simulink model "PMSMController"  (R2021a)
settings: Solver=FixedStepDiscrete  StartTime=0.0  StopTime=T_end  FixedStep=mask_Ts  RelTol=1e-3
values from neighbouring files (symbols this model uses):
  f_w = 50    [speedControlInit.m]
  Iq_max = 200    [speedControlInit.m]
  mask_Kaw = mask_Kis/mask_Kps    (= 1.25e-06)    [speedControlInit.m]
  mask_Kid = omega_ib*mask_R_s    (= 212.057504117)    [speedControlInit.m]
  mask_Kiq = omega_ib*mask_R_s    (= 212.057504117)    [speedControlInit.m]
  mask_Kis = omega_sb*B    (= 1.1780972451e-05)    [speedControlInit.m]
  mask_Kpd = omega_ib*mask_Ld    (= 0.249285377062)    [speedControlInit.m]
  mask_Kpq = omega_ib*mask_Lq    (= 0.249285377062)    [speedControlInit.m]
  mask_Kps = omega_sb*J    (= 9.42477796077)    [speedControlInit.m]
  mask_Kt = 0.126    [speedControlInit.m]
  mask_lambda_pm = mask_Kt/((3/2)*mask_p)    (= 0.0105)    [speedControlInit.m]
  mask_Ld = 52.9e-6    (= 5.29e-05)    [speedControlInit.m]
  mask_Lq = 52.9e-6    (= 5.29e-05)    [speedControlInit.m]
  mask_p = 8    [speedControlInit.m]
  mask_Ts = 1/10000    (= 0.0001)    [speedControlInit.m]
  mask_VDC = 250    [speedControlInit.m]
libraries: pid_lib x3
settings Model: Creator=Nishanth  LastModifiedBy=Nishanth
settings SolverCC: AlgebraicLoopSolver=TrustRegion
settings DataIOCC: SaveOutput=off  SaveTime=off
settings OptimizationCC: DefaultParameterBehavior=Inlined  EnhancedBackFolding=on  PassReuseOutputArgsAs=Individual arguments  ZeroExternalMemoryAtStartup=off  ZeroInternalMemoryAtStartup=off  NoFixptDivByZeroProtection=on  EfficientFloat2IntCast=on  OptimizeBlockOrder=speed  DifferentSizesBufferReuse=on  OptimizationCustomize=off  EfficientTunableParamExpr=on
settings DebuggingCC: ParameterTunabilityLossMsg=error  SFMachineParentedDataDiag=warning
settings SFSimCC: MATLABDynamicMemAlloc=off
settings RTWCC: SystemTargetFile=ert.tlc  GenCodeOnly=on  TemplateMakefile=ert_default_tmf  GenerateReport=on  LaunchReport=on  GenerateCodeMetricsReport=on
settings CodeAppCC: ForceParamTrailComments=on  IgnoreCustomStorageClasses=off  OperatorAnnotations=on  SimulinkDataObjDesc=on  SFDataObjDesc=on  InsertBlockDesc=on
settings ERTTargetCC: TargetLangStandard=C99 (ISO)  SupportNonFinite=off  RemoveResetFunc=off  InlinedParameterPlacement=NonHierarchical  ERTCustomFileTemplate=example_file_process.tlc

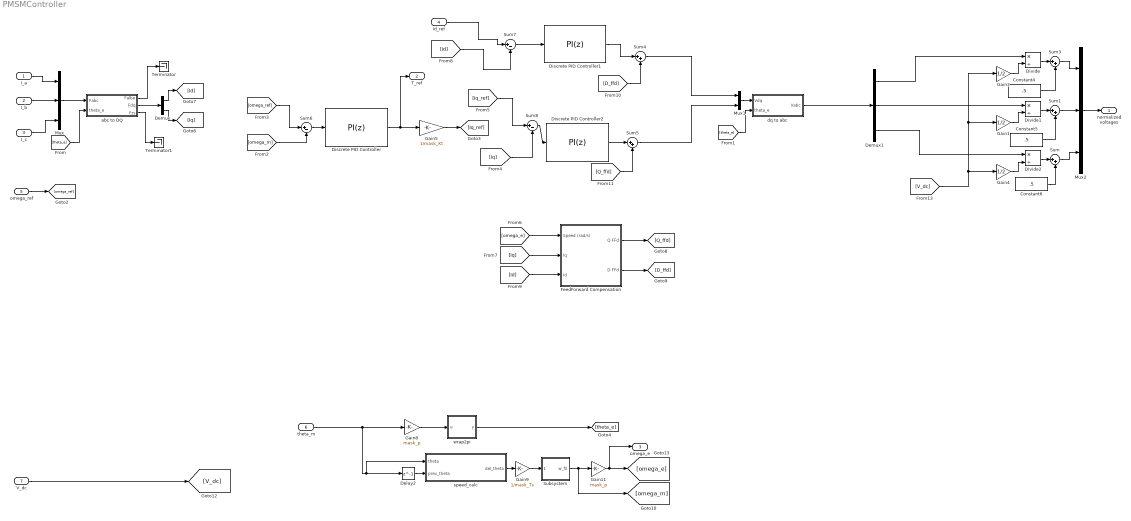
== system PMSMController ==
  I_a : Inport  OutDataTypeStr=double  PortDimensions=1
  I_b : Inport  Port=2  OutDataTypeStr=double  PortDimensions=1
  I_c : Inport  Port=3  OutDataTypeStr=double  PortDimensions=1
  Id_ref : Inport  Port=4  OutDataTypeStr=double  PortDimensions=1
  omega_ref : Inport  Port=5  OutDataTypeStr=double  PortDimensions=1
  theta_m : Inport  Port=6  OutDataTypeStr=double  PortDimensions=1
  V_dc : Inport  Port=7  OutDataTypeStr=double  PortDimensions=1
  Constant4 : Constant  Value=.5
  Constant5 : Constant  Value=.5
  Constant6 : Constant  Value=.5
  Delay2 : Delay  DelayLength=1
  Demux : Demux  Outputs=2
  Demux1 : Demux  Outputs=3
  Discrete PID Controller : pid_lib/PID Controller  Controller=PI  Form=Parallel  TimeDomain=Discrete-time  UseExternalTs=off  SampleTime=-1  IntegratorMethod=Forward Euler  FilterMethod=Forward Euler  ControllerParametersSource=internal  P=mask_Kps  I=mask_Kis  D=0  UseFilter=off  N=100  TunerSelectOption=Transfer Function Based (PID Tuner App)  ZeroCross=off  InitialConditionSource=internal  InitialConditionForIntegrator=0  InitialConditionForFilter=0  DifferentiatorICPrevScaledInput=0  ExternalReset=none  TrackingMode=off  Kt=1  LimitOutput=on  SatLimitsSource=internal  UpperSaturationLimit=Iq_max*mask_Kt  LowerSaturationLimit=-Iq_max*mask_Kt  LinearizeAsGain=off  AntiWindupMode=back-calculation  Kb=mask_Kaw  POutMin=[]  POutMax=[]  IOutMin=[]  IOutMax=[]  DOutMin=[]  DOutMax=[]  NOutMin=[]  NOutMax=[]  SumOutMin=[]  SumOutMax=[]  SaturationOutMin=[]  SaturationOutMax=[]  PParamMin=[]  PParamMax=[]  IParamMin=[]  IParamMax=[]  DParamMin=[]  DParamMax=[]  NParamMin=[]  NParamMax=[]  KbParamMin=[]  KbParamMax=[]  KtParamMin=[]  KtParamMax=[]  KbOutMin=[]  KbOutMax=[]  KtOutMin=[]  KtOutMax=[]  IntegratorOutMin=[]  IntegratorOutMax=[]  FilterOutMin=[]  FilterOutMax=[]  SumI1OutMin=[]  SumI1OutMax=[]  SumI2OutMin=[]  SumI2OutMax=[]  SumI3OutMin=[]  SumI3OutMax=[]  SumI4OutMin=[]  SumI4OutMax=[]  SumDOutMin=[]  SumDOutMax=[]  DifferentiatorOutMin=[]  DifferentiatorOutMax=[]  FilterDiffOutCoefMin=[]  FilterDiffOutCoefMax=[]  ReciprocalOutMin=[]  ReciprocalOutMax=[]  SumDenOutMin=[]  SumDenOutMax=[]  SumNumOutMin=[]  SumNumOutMax=[]  DivideOutMin=[]  DivideOutMax=[]  UdiffTsProdOutMin=[]  UdiffTsProdOutMax=[]  NTsProdOutMin=[]  NTsProdOutMax=[]  UintegralTsProdOutMin=[]  UintegralTsProdOutMax=[]  UngainTsProdOutMin=[]  UngainTsProdOutMax=[]  IntegratorContinuousStateAttributes=''  IntegratorStateMustResolveToSignalObject=off  IntegratorRTWStateStorageClass=Auto  FilterContinuousStateAttributes=''  FilterStateMustResolveToSignalObject=off  FilterRTWStateStorageClass=Auto  ParallelPVariant=InternalParameters  IdealPVariant=Disabled  IVariant=InternalParameters  DVariant=Disabled  IntegratorVariant=Discrete  SatVariant=Enabled  AWVariant=BackCalculation  PCopyVariant=Disabled  TRVariant=Disabled  FdbkBlocksVariant=Forward  IdealPFdbkVariant=Disabled  SatFdbkVariant=Disabled  DerivativeFilterVariant=Disabled  NVariant=Disabled  NCopyVariant=Disabled_SignalSpec  FilterICVariant=Disabled  IntegratorICVariant=InternalICs  ExternalResetVariant=Disabled  TRSumVariant=Passthrough  SumFdbkVariant=Disabled  SumVariant=Sum_PI  TsampFilterVariant=InternalTs  TsampNgainVariant=Passthrough  TsampIntegralVariant=Passthrough  ExternalSaturationOutDataTypeStr=Inherit: Same as second input
  Discrete PID Controller1 : pid_lib/PID Controller  Controller=PI  Form=Parallel  TimeDomain=Discrete-time  UseExternalTs=off  SampleTime=-1  IntegratorMethod=Forward Euler  FilterMethod=Forward Euler  ControllerParametersSource=internal  P=mask_Kpd  I=mask_Kid  D=0  UseFilter=off  N=100  TunerSelectOption=Transfer Function Based (PID Tuner App)  ZeroCross=off  InitialConditionSource=internal  InitialConditionForIntegrator=0  InitialConditionForFilter=0  DifferentiatorICPrevScaledInput=0  ExternalReset=none  TrackingMode=off  Kt=1  LimitOutput=off  SatLimitsSource=internal  UpperSaturationLimit=mask_VDC/2  LowerSaturationLimit=-mask_VDC/2  LinearizeAsGain=off  AntiWindupMode=back-calculation  Kb=mask_Kaw  POutMin=[]  POutMax=[]  IOutMin=[]  IOutMax=[]  DOutMin=[]  DOutMax=[]  NOutMin=[]  NOutMax=[]  SumOutMin=[]  SumOutMax=[]  SaturationOutMin=[]  SaturationOutMax=[]  PParamMin=[]  PParamMax=[]  IParamMin=[]  IParamMax=[]  DParamMin=[]  DParamMax=[]  NParamMin=[]  NParamMax=[]  KbParamMin=[]  KbParamMax=[]  KtParamMin=[]  KtParamMax=[]  KbOutMin=[]  KbOutMax=[]  KtOutMin=[]  KtOutMax=[]  IntegratorOutMin=[]  IntegratorOutMax=[]  FilterOutMin=[]  FilterOutMax=[]  SumI1OutMin=[]  SumI1OutMax=[]  SumI2OutMin=[]  SumI2OutMax=[]  SumI3OutMin=[]  SumI3OutMax=[]  SumI4OutMin=[]  SumI4OutMax=[]  SumDOutMin=[]  SumDOutMax=[]  DifferentiatorOutMin=[]  DifferentiatorOutMax=[]  FilterDiffOutCoefMin=[]  FilterDiffOutCoefMax=[]  ReciprocalOutMin=[]  ReciprocalOutMax=[]  SumDenOutMin=[]  SumDenOutMax=[]  SumNumOutMin=[]  SumNumOutMax=[]  DivideOutMin=[]  DivideOutMax=[]  UdiffTsProdOutMin=[]  UdiffTsProdOutMax=[]  NTsProdOutMin=[]  NTsProdOutMax=[]  UintegralTsProdOutMin=[]  UintegralTsProdOutMax=[]  UngainTsProdOutMin=[]  UngainTsProdOutMax=[]  IntegratorContinuousStateAttributes=''  IntegratorStateMustResolveToSignalObject=off  IntegratorRTWStateStorageClass=Auto  FilterContinuousStateAttributes=''  FilterStateMustResolveToSignalObject=off  FilterRTWStateStorageClass=Auto  ParallelPVariant=InternalParameters  IdealPVariant=Disabled  IVariant=InternalParameters  DVariant=Disabled  IntegratorVariant=Discrete  SatVariant=Disabled  AWVariant=Passthrough  PCopyVariant=Disabled  TRVariant=Disabled  FdbkBlocksVariant=Forward  IdealPFdbkVariant=Disabled  SatFdbkVariant=Disabled  DerivativeFilterVariant=Disabled  NVariant=Disabled  NCopyVariant=Disabled_SignalSpec  FilterICVariant=Disabled  IntegratorICVariant=InternalICs  ExternalResetVariant=Disabled  TRSumVariant=Passthrough  SumFdbkVariant=Disabled  SumVariant=Sum_PI  TsampFilterVariant=InternalTs  TsampNgainVariant=Passthrough  TsampIntegralVariant=Passthrough  ExternalSaturationOutDataTypeStr=Inherit: Same as second input
  Discrete PID Controller2 : pid_lib/PID Controller  Controller=PI  Form=Parallel  TimeDomain=Discrete-time  UseExternalTs=off  SampleTime=-1  IntegratorMethod=Forward Euler  FilterMethod=Forward Euler  ControllerParametersSource=internal  P=mask_Kpq  I=mask_Kiq  D=0  UseFilter=off  N=100  TunerSelectOption=Transfer Function Based (PID Tuner App)  ZeroCross=off  InitialConditionSource=internal  InitialConditionForIntegrator=0  InitialConditionForFilter=0  DifferentiatorICPrevScaledInput=0  ExternalReset=none  TrackingMode=off  Kt=1  LimitOutput=off  SatLimitsSource=internal  UpperSaturationLimit=mask_VDC/2  LowerSaturationLimit=-mask_VDC/2  LinearizeAsGain=off  AntiWindupMode=back-calculation  Kb=mask_Kaw  POutMin=[]  POutMax=[]  IOutMin=[]  IOutMax=[]  DOutMin=[]  DOutMax=[]  NOutMin=[]  NOutMax=[]  SumOutMin=[]  SumOutMax=[]  SaturationOutMin=[]  SaturationOutMax=[]  PParamMin=[]  PParamMax=[]  IParamMin=[]  IParamMax=[]  DParamMin=[]  DParamMax=[]  NParamMin=[]  NParamMax=[]  KbParamMin=[]  KbParamMax=[]  KtParamMin=[]  KtParamMax=[]  KbOutMin=[]  KbOutMax=[]  KtOutMin=[]  KtOutMax=[]  IntegratorOutMin=[]  IntegratorOutMax=[]  FilterOutMin=[]  FilterOutMax=[]  SumI1OutMin=[]  SumI1OutMax=[]  SumI2OutMin=[]  SumI2OutMax=[]  SumI3OutMin=[]  SumI3OutMax=[]  SumI4OutMin=[]  SumI4OutMax=[]  SumDOutMin=[]  SumDOutMax=[]  DifferentiatorOutMin=[]  DifferentiatorOutMax=[]  FilterDiffOutCoefMin=[]  FilterDiffOutCoefMax=[]  ReciprocalOutMin=[]  ReciprocalOutMax=[]  SumDenOutMin=[]  SumDenOutMax=[]  SumNumOutMin=[]  SumNumOutMax=[]  DivideOutMin=[]  DivideOutMax=[]  UdiffTsProdOutMin=[]  UdiffTsProdOutMax=[]  NTsProdOutMin=[]  NTsProdOutMax=[]  UintegralTsProdOutMin=[]  UintegralTsProdOutMax=[]  UngainTsProdOutMin=[]  UngainTsProdOutMax=[]  IntegratorContinuousStateAttributes=''  IntegratorStateMustResolveToSignalObject=off  IntegratorRTWStateStorageClass=Auto  FilterContinuousStateAttributes=''  FilterStateMustResolveToSignalObject=off  FilterRTWStateStorageClass=Auto  ParallelPVariant=InternalParameters  IdealPVariant=Disabled  IVariant=InternalParameters  DVariant=Disabled  IntegratorVariant=Discrete  SatVariant=Disabled  AWVariant=Passthrough  PCopyVariant=Disabled  TRVariant=Disabled  FdbkBlocksVariant=Forward  IdealPFdbkVariant=Disabled  SatFdbkVariant=Disabled  DerivativeFilterVariant=Disabled  NVariant=Disabled  NCopyVariant=Disabled_SignalSpec  FilterICVariant=Disabled  IntegratorICVariant=InternalICs  ExternalResetVariant=Disabled  TRSumVariant=Passthrough  SumFdbkVariant=Disabled  SumVariant=Sum_PI  TsampFilterVariant=InternalTs  TsampNgainVariant=Passthrough  TsampIntegralVariant=Passthrough  ExternalSaturationOutDataTypeStr=Inherit: Same as second input
  Divide : Product  Inputs=*/
  Divide1 : Product  Inputs=*/
  Divide2 : Product  Inputs=*/
  "FeedForward Compensation " : Subsystem
  Gain1 : Gain  Gain=1/2
  Gain11 : Gain  Gain=mask_p
  Gain3 : Gain  Gain=1/2
  Gain4 : Gain  Gain=1/2
  Gain5 : Gain  Gain=1/mask_Kt
  Gain8 : Gain  Gain=mask_p
  Gain9 : Gain  Gain=1/mask_Ts
  Mux : Mux  Inputs=3
  Mux1 : Mux  Inputs=2
  Mux2 : Mux  Inputs=3
  Subsystem : Subsystem
  Sum{,1,3..5} (5 alike) : Sum  Inputs=|++
  Sum6 : Sum  Inputs=|+-
  Sum7 : Sum  Inputs=|+-
  Sum8 : Sum  Inputs=|+-
  Terminator : Terminator
  Terminator1 : Terminator
  abc to DQ : Subsystem
  dq to abc : Subsystem
  speed_calc : MATLAB Function  TreatAsAtomicUnit=on
  wrap2pi : MATLAB Function  TreatAsAtomicUnit=on
  normalized voltages : Outport
  T_ref : Outport  Port=2
  omega_e : Outport  Port=3
  wires:
  I_b/1 -> Mux/2
  I_c/1 -> Mux/3
  I_a/1 -> Mux/1
  abc to DQ/2(Fdq) -> Demux/1
  [theta_e] -> dq to abc/2(theta_e)
  Mux1/1 -> dq to abc/1(Vdq)
  Id_ref/1 -> Sum7/1
  Mux/1 -> abc to DQ/1(Fabc)
  [theta_e] -> abc to DQ/2(theta_e)
  Demux1/3 -> Divide2/1
  Gain1/1 -> Divide1/2
  dq to abc/1(Vabc) -> Demux1/1
  Demux1/2 -> Divide1/1
  Gain3/1 -> Divide/2
  Demux1/1 -> Divide/1
  Gain4/1 -> Divide2/2
  [V_dc] -> Gain3/1, Gain1/1, Gain4/1
  Mux2/1 -> normalized voltages/1
  Divide/1 -> Sum3/1
  Divide2/1 -> Sum/1
  Divide1/1 -> Sum1/1
  Sum/1 -> Mux2/3
  Sum1/1 -> Mux2/2
  Sum3/1 -> Mux2/1
  Constant4/1 -> Sum3/2
  Constant5/1 -> Sum1/2
  Constant6/1 -> Sum/2
  omega_ref/1 -> [omega_ref]
  [omega_ref] -> Sum6/1
  [omega_m] -> Sum6/2
  Discrete PID Controller/1 -> T_ref/1, Gain5/1
  Demux/2 -> [Iq]
  [Iq] -> Sum8/2
  [omega_e] -> "FeedForward Compensation "/1(Speed (rad/s))
  [Iq] -> "FeedForward Compensation "/2(Iq)
  [Id] -> Sum7/2
  Demux/1 -> [Id]
  [Id] -> "FeedForward Compensation "/3(Id)
  "FeedForward Compensation "/1(Q FFd) -> [Q_ffd]
  "FeedForward Compensation "/2(D FFd) -> [D_ffd]
  Discrete PID Controller2/1 -> Sum5/1
  Sum4/1 -> Mux1/1
  Sum5/1 -> Mux1/2
  [Q_ffd] -> Sum5/2
  [D_ffd] -> Sum4/2
  V_dc/1 -> [V_dc]
  Sum6/1 -> Discrete PID Controller/1
  Gain5/1 -> [Iq_ref]
  Sum7/1 -> Discrete PID Controller1/1
  Discrete PID Controller1/1 -> Sum4/1
  Sum8/1 -> Discrete PID Controller2/1
  [Iq_ref] -> Sum8/1
  abc to DQ/1(Falbe) -> Terminator/1
  abc to DQ/3(Fzs) -> Terminator1/1
  Gain8/1 -> wrap2pi/1(u)
  Gain11/1 -> [omega_e], omega_e/1
  speed_calc/1(del_theta) -> Gain9/1
  Gain9/1 -> Subsystem/1(omega)
  Subsystem/1(w_fil) -> [omega_m], Gain11/1
  Delay2/1 -> speed_calc/2(prev_theta)
  wrap2pi/1(y) -> [theta_e]
  theta_m/1 -> speed_calc/1(theta), Delay2/1, Gain8/1

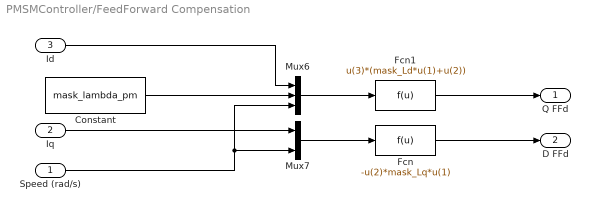
== system PMSMController/FeedForward Compensation  ==
  Speed (rad/s) : Inport
  Iq : Inport  Port=2
  Id : Inport  Port=3
  Constant : Constant  Value=mask_lambda_pm  SampleTime=-1
  Fcn : Fcn  Expr=-u(2)*mask_Lq*u(1)
  Fcn1 : Fcn  Expr=u(3)*(mask_Ld*u(1)+u(2))
  Mux6 : Mux  Inputs=3
  Mux7 : Mux  Inputs=2
  Q FFd : Outport  VectorParamsAs1DForOutWhenUnconnected=off
  D FFd : Outport  Port=2  VectorParamsAs1DForOutWhenUnconnected=off
  wires:
  Constant/1 -> Mux6/2
  Fcn1/1 -> Q FFd/1
  Fcn/1 -> D FFd/1
  Speed (rad/s)/1 -> Mux7/2, Mux6/3
  Iq/1 -> Mux7/1
  Id/1 -> Mux6/1
  Mux6/1 -> Fcn1/1
  Mux7/1 -> Fcn/1

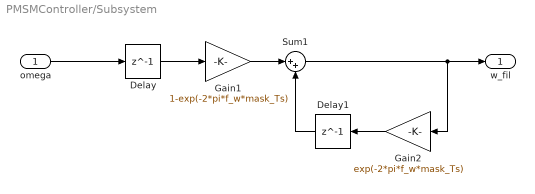
== system PMSMController/Subsystem ==
  omega : Inport
  Delay : Delay  DelayLength=1
  Delay1 : Delay  DelayLength=1
  Gain1 : Gain  Gain=1-exp(-2*pi*f_w*mask_Ts)
  Gain2 : Gain  Gain=exp(-2*pi*f_w*mask_Ts)
  Sum1 : Sum  Inputs=|++
  w_fil : Outport
  wires:
  Delay/1 -> Gain1/1
  omega/1 -> Delay/1
  Gain1/1 -> Sum1/1
  Sum1/1 -> Gain2/1, w_fil/1
  Delay1/1 -> Sum1/2
  Gain2/1 -> Delay1/1

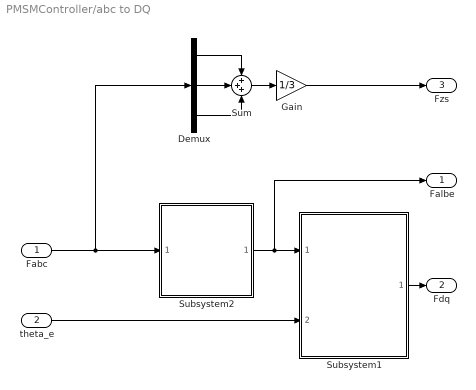
== system PMSMController/abc to DQ ==
  Fabc : Inport
  theta_e : Inport  Port=2
  Demux : Demux  Outputs=3
  Gain : Gain  Gain=1/3
  Subsystem1 : Subsystem  ReferencedSubsystem=Falphabeta_to_Fdq
  Subsystem2 : Subsystem  ReferencedSubsystem=F3ph_to_F2ph
  Sum : Sum  Inputs=+++
  Falbe : Outport
  Fdq : Outport  Port=2
  Fzs : Outport  Port=3  PortDimensions=1
  wires:
  Gain/1 -> Fzs/1
  Demux/2 -> Sum/2
  Sum/1 -> Gain/1
  theta_e/1 -> Subsystem1/2
  Demux/1 -> Sum/1
  Demux/3 -> Sum/3
  Fabc/1 -> Subsystem2/1, Demux/1
  Subsystem2/1 -> Subsystem1/1, Falbe/1
  Subsystem1/1 -> Fdq/1

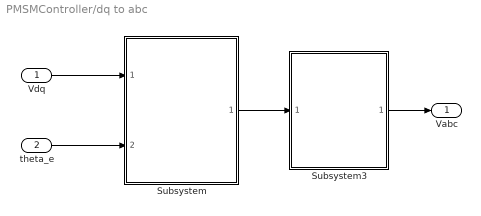
== system PMSMController/dq to abc ==
  Vdq : Inport  PortDimensions=2
  theta_e : Inport  Port=2  PortDimensions=1
  Subsystem : Subsystem  ReferencedSubsystem=Fdq_to_Falphabeta
  Subsystem3 : Subsystem  ReferencedSubsystem=F2ph_to_F3ph
  Vabc : Outport  PortDimensions=3
  wires:
  theta_e/1 -> Subsystem/2
  Subsystem/1 -> Subsystem3/1
  Vdq/1 -> Subsystem/1
  Subsystem3/1 -> Vabc/1

== matlab function PMSMController/speed_calc ==
  data: theta input; del_theta output; prev_theta input
function del_theta = delta_theta(theta, prev_theta)

    % check if prev_theta exist before using to prevent error in 1st iteration 
    del_theta = theta - prev_theta;

    % prevent jumps in speed during 2pi to 0 transitions 
    while del_theta > pi
        del_theta = del_theta - 2*pi;
    end

    while del_theta < -pi
        del_theta = del_theta + 2*pi;
    end
    
end

== matlab function PMSMController/wrap2pi ==
  data: u input; y output
function y = wrap2pi(u)

y = u;

while y > 2*pi
    y = y - 2*pi;
end

while y < 0
    y = y + 2*pi;
end

end
